simulink model "ship_Path_round"  (Simulink 8.4)
settings: Solver=ode5  StartTime=0.0  StopTime=2000  FixedStep=0.1  RelTol=1e-3
libraries: simulink x1
settings Model: Creator=Administrator  LastModifiedBy=Yifang
settings SolverCC: ZeroCrossControl=DisableAll
settings DebuggingCC: FcnCallInpInsideContextMsg=EnableAllAsError  FrameProcessingCompatibilityMsg=error
settings ConfigComp: CovMetricSettings=dw  CovHtmlReporting=on  CovSaveCumulativeToWorkspaceVar=on  CovSaveSingleToWorkspaceVar=on  CovExternalEMLEnable=off  CovSFcnEnable=off

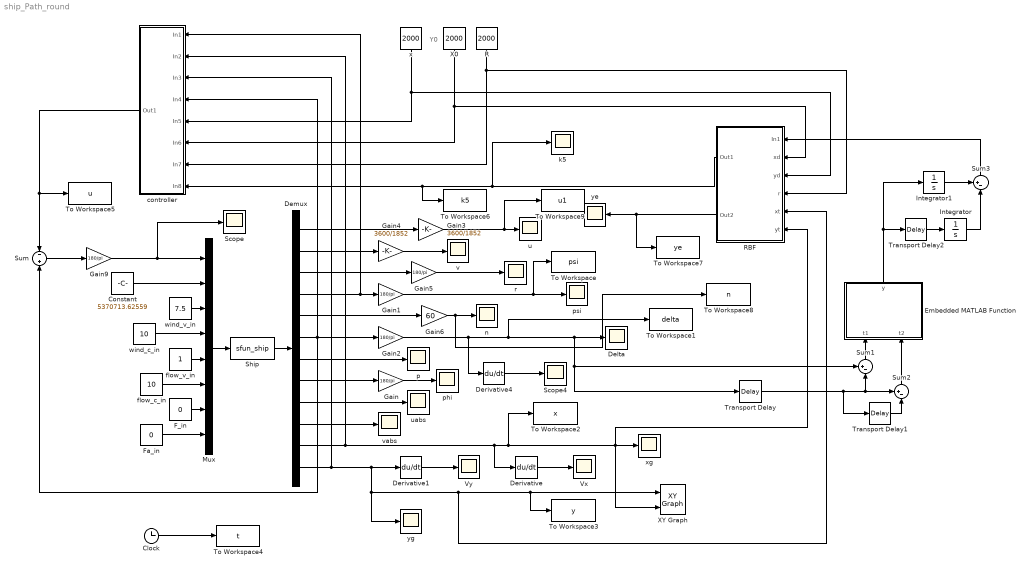
== system ship_Path_round ==
  note: Y0
  Clock : Clock
  Constant : Constant  Value=5370713.62559
  Delta : Scope
  Demux : Demux  Outputs=12
  Derivative : Derivative
  Derivative1 : Derivative
  Derivative4 : Derivative
  Embedded MATLAB Function : MATLAB Function  TreatAsAtomicUnit=on
  F_in : Constant  Value=0
  Fa_in : Constant  Value=0
  Gain{,1..2,5,9} (5 alike) : Gain  Gain=180/pi
  Gain3 : Gain  Gain=3600/1852
  Gain4 : Gain  Gain=3600/1852
  Gain6 : Gain  Gain=60
  Integrator : Integrator
  Integrator1 : Integrator
  Mux : Mux  Inputs=8
  R : Constant  Value=2000
  RBF : Subsystem
  Scope : Scope
  Scope4 : Scope
  Ship : S-Function  FunctionName=sfun_ship  EnableBusSupport=off
  Sum : Sum  Inputs=-|+
  Sum1 : Sum  Inputs=+-|
  Sum2 : Sum  Inputs=+-|
  Sum3 : Sum  Inputs=+-|
  To Workspace : ToWorkspace  VariableName=psi  SampleTime=-1
  To Workspace1 : ToWorkspace  VariableName=delta  SampleTime=-1
  To Workspace2 : ToWorkspace  VariableName=x  SampleTime=-1
  To Workspace3 : ToWorkspace  VariableName=y  SampleTime=-1
  To Workspace4 : ToWorkspace  VariableName=t  SampleTime=-1
  To Workspace5 : ToWorkspace  VariableName=u  SampleTime=-1
  To Workspace6 : ToWorkspace  VariableName=k5  SampleTime=-1
  To Workspace7 : ToWorkspace  VariableName=ye  SampleTime=-1
  To Workspace8 : ToWorkspace  VariableName=n  SampleTime=-1
  To Workspace9 : ToWorkspace  VariableName=u1  SampleTime=-1
  Transport Delay : TransportDelay
  Transport Delay1 : TransportDelay
  Transport Delay2 : TransportDelay  DelayTime=50
  Vx : Scope
  Vy : Scope
  X0 : Constant  Value=2000
  XY Graph : simulink/Sinks/XY Graph  xmin=-1500  xmax=5000  ymin=-1500  ymax=5000  st=-1
  controller : Subsystem
  flow_c_in : Constant  Value=10
  flow_v_in : Constant
  k5 : Scope
  n : Scope
  p : Scope
  phi : Scope
  psi : Scope
  r : Scope
  u : Scope
  uabs : Scope
  v : Scope
  vabs : Scope
  wind_c_in : Constant  Value=10
  wind_v_in : Constant  Value=7.5
  x : Constant  Value=2000
  xg : Scope
  ye : Scope
      settings: TickLabels=on  TimeRange=800  YMin=-110.20471  YMax=932.71955  SaveName=delta3
  yg : Scope
  wires:
  Ship/1 -> Demux/1
  Demux/1 -> Gain3/1
  Demux/2 -> Gain4/1
  Demux/3 -> Gain5/1
  Demux/5 -> Gain6/1
  Demux/7 -> p/1
  Demux/8 -> Gain/1
  Gain1/1 -> psi/1, To Workspace/1
  Gain/1 -> phi/1
  Gain3/1 -> u/1, To Workspace9/1
  Gain4/1 -> v/1
  Gain5/1 -> r/1
  Gain6/1 -> To Workspace8/1, n/1
  Demux/9 -> uabs/1
  Demux/10 -> vabs/1
  Demux/12 -> Derivative1/1, yg/1, To Workspace3/1, XY Graph/1, RBF/5(xt), controller/3(In3)
  Demux/11 -> Derivative/1, To Workspace2/1, RBF/6(yt), XY Graph/2, xg/1, controller/2(In2)
  wind_v_in/1 -> Mux/3
  wind_c_in/1 -> Mux/4
  flow_v_in/1 -> Mux/5
  F_in/1 -> Mux/7
  Fa_in/1 -> Mux/8
  flow_c_in/1 -> Mux/6
  Mux/1 -> Ship/1
  Constant/1 -> Mux/2
  Sum/1 -> Gain9/1
  Derivative4/1 -> Scope4/1
  controller/1(Out1) -> Sum/1, To Workspace5/1
  Demux/4 -> controller/1(In1), Gain1/1
  Gain2/1 -> Derivative4/1, To Workspace1/1, Transport Delay/1, Sum1/1, Delta/1
  Gain9/1 -> Mux/1, Scope/1
  Clock/1 -> To Workspace4/1
  x/1 -> controller/5(In5), RBF/3(yd)
  X0/1 -> controller/6(In6), RBF/2(xd)
  R/1 -> controller/7(In7), RBF/4(r)
  Transport Delay/1 -> Sum1/2, Sum2/1, Transport Delay1/1
  Sum1/1 -> Embedded MATLAB Function/1(t1)
  Transport Delay1/1 -> Sum2/2
  Sum2/1 -> Embedded MATLAB Function/2(t2)
  Embedded MATLAB Function/1(y) -> Transport Delay2/1, Integrator1/1
  Transport Delay2/1 -> Integrator/1
  Integrator1/1 -> Sum3/1
  Integrator/1 -> Sum3/2
  Sum3/1 -> RBF/1(In1)
  Derivative1/1 -> Vy/1
  Derivative/1 -> Vx/1
  Demux/6 -> Gain2/1, Sum/2, controller/4(In4)
  RBF/2(Out2) -> To Workspace7/1, ye/1
  RBF/1(Out1) -> k5/1, controller/8(In8), To Workspace6/1

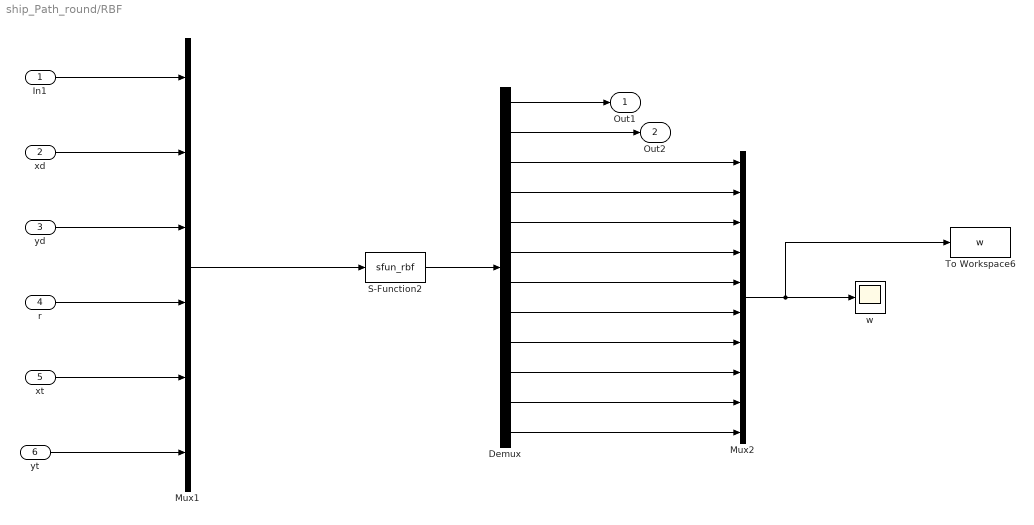
== system ship_Path_round/RBF ==
  In1 : Inport
  xd : Inport  Port=2
  yd : Inport  Port=3
  r : Inport  Port=4
  xt : Inport  Port=5
  yt : Inport  Port=6
  Demux : Demux  Outputs=12
  Mux1 : Mux  Inputs=6
  Mux2 : Mux  Inputs=10
  S-Function2 : S-Function  FunctionName=sfun_rbf  EnableBusSupport=off
  To Workspace6 : ToWorkspace  VariableName=w  SampleTime=-1
  w : Scope
  Out1 : Outport
  Out2 : Outport  Port=2
  wires:
  In1/1 -> Mux1/1
  xd/1 -> Mux1/2
  yd/1 -> Mux1/3
  r/1 -> Mux1/4
  xt/1 -> Mux1/5
  yt/1 -> Mux1/6
  S-Function2/1 -> Demux/1
  Demux/1 -> Out1/1
  Demux/2 -> Out2/1
  Mux1/1 -> S-Function2/1
  Demux/3 -> Mux2/1
  Demux/4 -> Mux2/2
  Demux/5 -> Mux2/3
  Demux/6 -> Mux2/4
  Demux/7 -> Mux2/5
  Demux/8 -> Mux2/6
  Demux/9 -> Mux2/7
  Demux/10 -> Mux2/8
  Demux/11 -> Mux2/9
  Demux/12 -> Mux2/10
  Mux2/1 -> To Workspace6/1, w/1

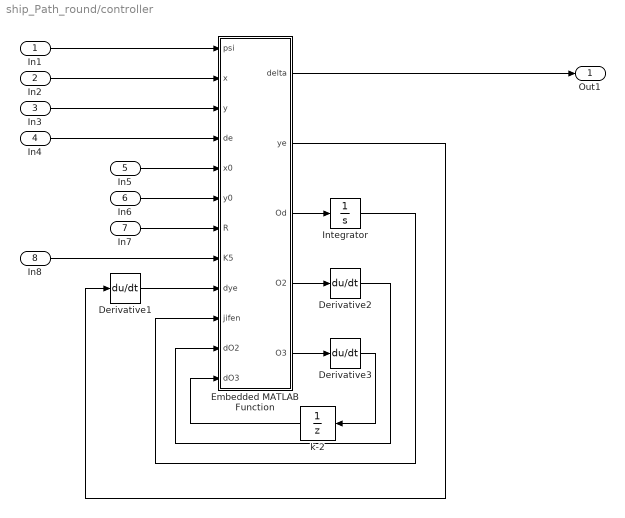
== system ship_Path_round/controller ==
  In1 : Inport
  In2 : Inport  Port=2
  In3 : Inport  Port=3
  In4 : Inport  Port=4
  In5 : Inport  Port=5
  In6 : Inport  Port=6
  In7 : Inport  Port=7
  In8 : Inport  Port=8
  Derivative1 : Derivative
  Derivative2 : Derivative
  Derivative3 : Derivative
  Embedded MATLAB Function : MATLAB Function  TreatAsAtomicUnit=on
  Integrator : Integrator
  k-2 : UnitDelay  SampleTime=-1
  Out1 : Outport
  wires:
  Embedded MATLAB Function/5(O3) -> Derivative3/1
  Derivative3/1 -> k-2/1
  Embedded MATLAB Function/4(O2) -> Derivative2/1
  Derivative2/1 -> Embedded MATLAB Function/11(dO2)
  Integrator/1 -> Embedded MATLAB Function/10(jifen)
  Embedded MATLAB Function/1(delta) -> Out1/1
  Embedded MATLAB Function/3(Od) -> Integrator/1
  In1/1 -> Embedded MATLAB Function/1(psi)
  In2/1 -> Embedded MATLAB Function/2(x)
  In3/1 -> Embedded MATLAB Function/3(y)
  Derivative1/1 -> Embedded MATLAB Function/9(dye)
  Embedded MATLAB Function/2(ye) -> Derivative1/1
  In4/1 -> Embedded MATLAB Function/4(de)
  In5/1 -> Embedded MATLAB Function/5(x0)
  In6/1 -> Embedded MATLAB Function/6(y0)
  In7/1 -> Embedded MATLAB Function/7(R)
  In8/1 -> Embedded MATLAB Function/8(K5)
  k-2/1 -> Embedded MATLAB Function/12(dO3)

== matlab function Embedded MATLAB Function ==
  data: t1 input double; y output double; t2 input double
function y = fcn(t1,t2)
%#eml
if(t1*t2>0)
  p=0;
else
    p=1;
end
y = p*t1;

== matlab function controller/Embedded MATLAB Function ==
  data: psi input double; x input double; y input double; de input double; x0 input double; y0 input double; R input double; K5 input double; dye input double; delta output double; ye output double; Od output double; O2 output double; O3 output double; jifen input double; dO2 input double; dO3 input double
function [delta,ye,Od,O2,O3] = fcn(psi,x,y,de,x0,y0,R,K5,dye,jifen,dO2,dO3)
K0=0.01;K1=3;K2=0.05;K3=0.005;K4=0.01;
Te=2.5;%K5=3;

ye=sqrt((x-x0)^2+(y-y0)^2)-R;
if(de>0)
    psie=psi-atan2((y-y0),(x-x0))-pi/2;
else
    psie=psi-atan2((y-y0),(x-x0))+pi/2;
end


O1=K1*f(K0*ye)+dye;
Od=f(O1);
O2=psie+K2*jifen;
O3=K3*f(O2)+dO2;
O4=K4*f(O3)+dO3;
delta=-Te*K5*O4;
 function mean=f(a)
  mean=tanh(a);
%  function mean=f(a)
%  if(a<0.1&&a>-0.1)
%      mean=a;
%  else
%      mean=coth(a)-1/a;
%  end
